simulink model "rlwatertank_model2"  (R2020b)
settings: Solver=ode45  StartTime=0.0  StopTime=inf  RelTol=1e-3  EnableMultiTasking=on
undefined symbols (not defined in the file): DiscIntNeverNeededParam, Ts
libraries: simulink x2, rllib x1
settings Model: Creator=The MathWorks, Inc.  LastModifiedBy=Asus
settings DataIOCC: LimitDataPoints=on  SaveFormat=Array  SignalLoggingName=logsOut
settings OptimizationCC: ExpressionDepthLimit=2147483647  InitFltsAndDblsToZero=on  LifeSpan=inf
settings DebuggingCC: SaveWithParameterizedLinksMsg=none  UnderspecifiedInitializationDetection=Classic  MergeDetectMultiDrivingBlocksExec=none  SignalResolutionControl=TryResolveAllWithWarning  MultiTaskDSMMsg=warning  FcnCallInpInsideContextMsg=warning  AllowSymbolicDim=off  StateNameClashWarn=warning  SFUnexpectedBacktrackingDiag=warning  SFNoUnconditionalDefaultTransitionDiag=warning  SFExecutionAtInitializationDiag=none  ArithmeticOperatorsInVariantConditions=warning
settings HardwareCC: ProdBitPerPointer=32  ProdBitPerSizeT=32  ProdBitPerPtrDiffT=32  ProdLargestAtomicFloat=None  ProdIntDivRoundTo=Undefined  ProdEndianess=Unspecified  ProdWordSize=32  ProdHWDeviceType=Specified
settings ModelReferenceCC: PropagateSignalLabelsOutOfModel=off
settings SFSimCC: SimUseLocalCustomCode=off  CustomCodeUndefinedFunction=UseInterfaceOnly
settings RTWCC: RTWUseLocalCustomCode=off
settings CodeAppCC: StateflowObjectComments=on
settings GRTTargetCC: TargetFcnLib=ansi_tfl_tmw.mat  TargetLangStandard=C89/C90 (ANSI)  CombineOutputUpdateFcns=off  GRTInterface=on
settings ConfigComp: CovMetricSettings=dw  CovSaveCumulativeToWorkspaceVar=on  CovSaveSingleToWorkspaceVar=on  CovExternalEMLEnable=off

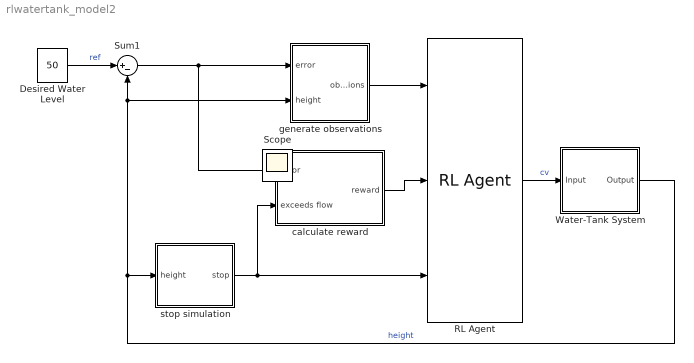
== system rlwatertank_model2 ==
  Desired Water Level : Constant  Value=50
  RL Agent : rllib/RL Agent  Agent=agent  ProvideReward=on  ProvideIsDone=on  ProvideCumRwd=off  TreatAsDirectFeedthrough=on  CollectLoggedSignals=on  CollectModelStates=on
      settings: SourceProductName=Reinforcement Learning
  Sum1 : Sum  Inputs=|+-  SaturateOnIntegerOverflow=on
  Water-Tank System : Subsystem
  calculate reward : Subsystem
  generate observations : Subsystem
  stop simulation : Subsystem
  Scope : Scope
  wires:
  Desired Water Level/1 -> Sum1/1  "ref"
  Sum1/1 -> calculate reward/1(error), generate observations/1(error)
  Water-Tank System/1(Output) -> stop simulation/1(height), generate observations/2(height), Sum1/2  "height"
  RL Agent/1 -> Water-Tank System/1(Input)  "cv"
  stop simulation/1(stop) -> calculate reward/2(exceeds flow), RL Agent/3
  generate observations/1(observations) -> RL Agent/1
  calculate reward/1(reward) -> RL Agent/2

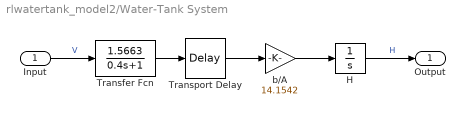
== system rlwatertank_model2/Water-Tank System ==
  Input : Inport
  H : Integrator  LimitOutput=on  LowerSaturationLimit=0
  Transfer Fcn : TransferFcn  Numerator=[1.5663]  Denominator=[0.4 1]
  Transport Delay : TransportDelay  DelayTime=0.3
  b/A : Gain  Gain=14.1542  SaturateOnIntegerOverflow=on  OutDataTypeStr=Inherit: Same as input  ParamDataTypeStr=Inherit: Same as input
  Output : Outport  VectorParamsAs1DForOutWhenUnconnected=off
  wires:
  H/1 -> Output/1  "H"
  Input/1 -> Transfer Fcn/1  "V"
  Transfer Fcn/1 -> Transport Delay/1
  Transport Delay/1 -> b/A/1
  b/A/1 -> H/1

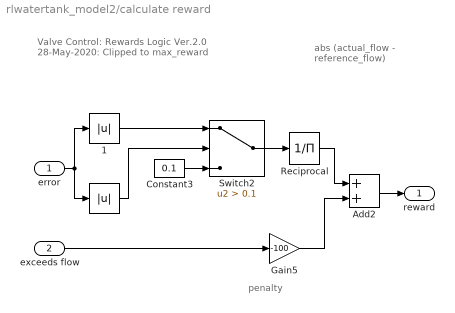
== system rlwatertank_model2/calculate reward ==
  note: penalty
  note: Valve Control: Rewards Logic
      | Ver.2.0 28-May-2020: Clipped to max_reward
  note: abs (actual_flow - reference_flow)
  error : Inport
  exceeds flow : Inport  Port=2
  " " : Abs
  " 1" : Abs
  Add2 : Sum
  Constant3 : Constant  Value=0.1
  Gain5 : Gain  Gain=-100
  Reciprocal : Product  Inputs=/
  Switch2 : Switch  Criteria=u2 > Threshold  Threshold=0.1
  reward : Outport  VectorParamsAs1DForOutWhenUnconnected=off
  wires:
  Constant3/1 -> Switch2/3
  Reciprocal/1 -> Add2/1
  Gain5/1 -> Add2/2
  " "/1 -> Switch2/2
  Switch2/1 -> Reciprocal/1
  Add2/1 -> reward/1
  " 1"/1 -> Switch2/1
  error/1 -> " 1"/1, " "/1
  exceeds flow/1 -> Gain5/1

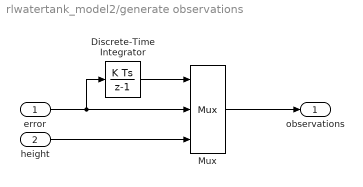
== system rlwatertank_model2/generate observations ==
  error : Inport
  height : Inport  Port=2
  Discrete-Time Integrator : DiscreteIntegrator  SampleTime=Ts  ICPrevOutput=DiscIntNeverNeededParam  ICPrevScaledInput=DiscIntNeverNeededParam
  Mux : Mux  Inputs=3
  observations : Outport  VectorParamsAs1DForOutWhenUnconnected=off
  wires:
  height/1 -> Mux/3
  Discrete-Time Integrator/1 -> Mux/1
  error/1 -> Discrete-Time Integrator/1, Mux/2
  Mux/1 -> observations/1

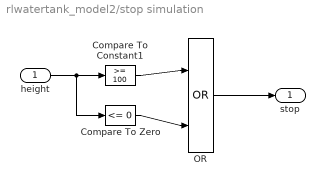
== system rlwatertank_model2/stop simulation ==
  height : Inport
  Compare To Constant1 : simulink/Logic and Bit Operations/Compare To Constant  relop=>=  const=100  OutDataTypeStr=boolean
  Compare To Zero : simulink/Logic and Bit Operations/Compare To Zero  relop=<=  OutDataTypeStr=boolean
  OR : Logic  Operator=OR  IconShape=distinctive  AllPortsSameDT=off  OutDataTypeStr=boolean
  stop : Outport  VectorParamsAs1DForOutWhenUnconnected=off
  wires:
  height/1 -> Compare To Zero/1, Compare To Constant1/1
  Compare To Zero/1 -> OR/2
  Compare To Constant1/1 -> OR/1
  OR/1 -> stop/1
